simulink model "ProjectOnSimulink__2_"  (R2022b)
settings: Solver=VariableStepAuto  StartTime=0.0  StopTime=10.0  RelTol=1e-3
undefined symbols (not defined in the file or in its folder): hw
libraries: raspberrypiAVlib x2
settings Model: Creator=mluser  LastModifiedBy=mluser

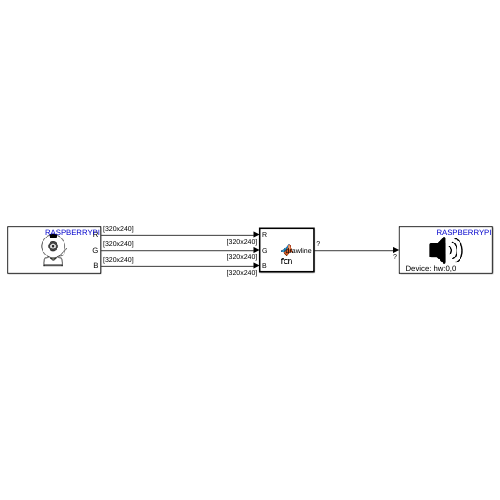
[thumbnail: Simulink's stored preview of the top-level diagram]
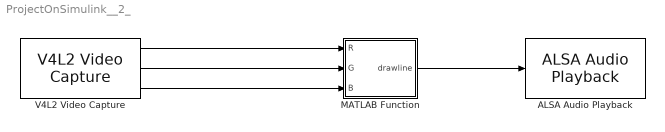
== system ProjectOnSimulink__2_ ==
  ALSA Audio Playback : raspberrypiAVlib/ALSA Audio Playback  deviceStr=hw:0,0  sampleRateEnum=44100  queueDuration=0.5  blockPlatform=LINUX
  MATLAB Function : MATLAB Function  TreatAsAtomicUnit=on
  V4L2 Video Capture : raspberrypiAVlib/V4L2 Video Capture  DeviceName=/dev/video0  Resolution=320x240  CustomResolution=[ 320, 240 ]  PixelFormat=RGB  SampleTime=0.1  pixelOrder=planar  simOutput=Colorbars  imSizeSelection=320x240  imSize=[640, 480]  roi=[0, 0, 640, 480]  m_devName='/dev/video0'  blockPlatform=LINUX  HorizontalFlip=off  VerticalFlip=off  Brightness=0.5  Saturation=0.5  Contrast=0.5  Sharpness=0.5  CameraPan=0  CameraTilt=0  CameraZoom=0.5  EnableManualFocus=on  ManualFocus=0.5
  wires:
  V4L2 Video Capture/1 -> MATLAB Function/1(R)
  MATLAB Function/1(drawline) -> ALSA Audio Playback/1
  V4L2 Video Capture/3 -> MATLAB Function/3(B)
  V4L2 Video Capture/2 -> MATLAB Function/2(G)

== matlab function ProjectOnSimulink__2_/MATLAB Function ==
  data: R input; G input; B input; drawline output
function drawline = fcn(R,G,B)  
im=cat(3,R,G,B); %%reconstitution de l'image
ini=rgb2gray(im);%%convertir l'image en niveaux de gris
l=imresize(ini,1/8);    %%compression
s=imsharpen(l);     %%sharpening the image
smo=imgaussfilt(s,5);   %%lissage de l'image

m=edge(smo,'log');%edges
n=size(l,1);
m=size(l,2);

for i=(1:n)
    p=0;%second limit
    j=0;%colonnes
    c=0;%compteur
    while(j<m)&&(c<2)
        j=j+1;
        if l(i,j)==1%si on trouve la première limite
            c=c+1;%on incrémente le compteur
            if c==2
                q=floor((p+j)/2);%q=milieu de la grande ligne
                l(i,q)=1;%tracage de la ligne
            end
            p=j;
        end
        
    end
end
%on se positionne au milieu à la dixième partie de l'image
a=round(n*9/10);
b=round(m/2);
%si on ne s'intéresse qu'à cette dernière partie ,la boucle qu'on vient de faire pour tracer le miliieu , pn peut la remplacer en se limitant  
%qu'à cette dernière partie qui nous interésse
lim=[];
for i=(1:m)
    if l(a,i)==1
        lim(end+1)=i;
    end
end
disp(lim);%lim contient les deux limites et le point de milieu qu'on vient de tracer%
l(a,b)=1;%position de l'utilisateur


Fs=44100;%fréquence

if (lim(2)<b) % l'utilisateur se trouve à droite
    Fs=44100;
    t=linspace(0,Fs*2,Fs*2);
    s=sin(2*pi*t*1000);
    Out=[zeros(size(t));s]';

    Volume=b-lim(2);
    s=s .*Volume;
    Out=[zeros(size(t));s]';
    sount(Out,Fs);

end

if (b<lim(2))  %% l'utilisateur se trouve à gauche
    t=linspace(0,Fs*2,Fs*2);
    s=sin(2*pi*t*1000);
    Volume = lim(2)-lim(b);
    s= s .*Volume;
    Out=[s;zeros(size(t))];
end

drawline=Out;
end
